simulink model "fboard_dwgn"  (Simulink 6.2)
settings: Solver=FixedStepDiscrete  SolverMode=SingleTasking  StartTime=0.0  StopTime=10.0  FixedStep=1  RelTol=1e-3
undefined symbols (not defined in the file): quant
libraries: xbsIndex_r3 x212, fb_xaui x1
(part 2 of 2)

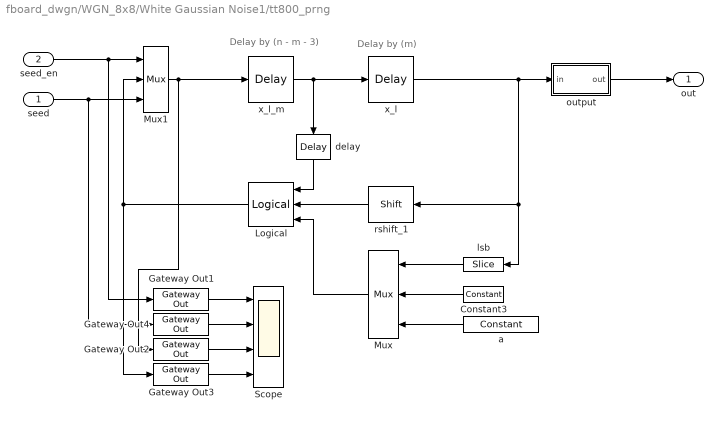
== system fboard_dwgn/WGN_8x8/White Gaussian Noise1/tt800_prng ==
  note: Delay by (n - m - 3)
  note: Delay by (m)
  seed : Inport  Port=1  LatchInput=off
  seed_en : Inport  Port=2  LatchInput=off
  Constant3 : xbsIndex_r3/Constant  Orientation=left  const=0  equ=P=C  arith_type=Unsigned  n_bits=32  bin_pt=0  opselect=C  inp2=PCIN>>17  opr=+  inp1=P  carry=CIN  iostate=0  explicit_period=off  period=1  dbl_ovrd=off
  Gateway Out{1..4} (4 alike) : xbsIndex_r3/Gateway Out  output_type=Double  nbits=8  bin_pt=6  arith_type=Boolean  quantization=Truncate  overflow=Wrap  hdl_port=off  timing_constraint=None  locs_specified=off  LOCs={}  needs_fixed_name=off  show_param=off
      settings: xl_area=[0 0 0 0 0 0 0]
  Logical : xbsIndex_r3/Logical  Orientation=left  logical_function=XOR  inputs=3  precision=Full  arith_type=Unsigned  n_bits=8  bin_pt=2  align_bp=off  latency=1  explicit_period=off  period=1  en=off  dbl_ovrd=off  show_param=on
      settings: xl_area=[32 32 0 32 0 0 0]
  Mux : xbsIndex_r3/Mux  Orientation=left  inputs=2  precision=Full  arith_type="Signed  (2's comp)"  n_bits=8  bin_pt=2  quantization=Truncate  overflow=Wrap  latency=1  explicit_period=off  period=1  en=off  dbl_ovrd=off  show_param=off  mux_type=off  use_rpm=off  gen_core=off
      settings: xl_area=[16 32 0 32 0 0 0]
  Mux1 : xbsIndex_r3/Mux  inputs=2  precision=Full  arith_type="Signed  (2's comp)"  n_bits=8  bin_pt=2  quantization=Truncate  overflow=Wrap  latency=1  explicit_period=on  period=1  en=off  dbl_ovrd=off  show_param=on  mux_type=off  use_rpm=off  gen_core=off
      settings: xl_area=[16 32 0 32 0 0 0]
  Scope : Scope  NumInputPorts=4
      settings: YMin=-5~-5~-5~-5  YMax=5~5~5~5
  a : xbsIndex_r3/Constant  Orientation=left  const=hex2dec('8EBFD028')  equ=P=C  arith_type=Unsigned  n_bits=32  bin_pt=0  opselect=C  inp2=PCIN>>17  opr=+  inp1=P  carry=CIN  iostate=0  explicit_period=off  period=1  dbl_ovrd=off
  delay : xbsIndex_r3/Delay  Orientation=down  latency=1  reg_retiming=off  explicit_period=off  period=1  en=off  accept_only_valid=off  init_zero=on  dbl_ovrd=off  show_param=off
      settings: xl_area=[16 32 0 0 0 0 0]
  lsb : xbsIndex_r3/Slice  Orientation=left  mode=Lower Bit Location + Width  nbits=1  bit1=0  base1=MSB of Input  bit0=0  base0=LSB of Input  boolean_output=off  explicit_period=off  period=1  dbl_ovrd=off
  output : Subsystem
  rshift_1 : xbsIndex_r3/Shift  Orientation=left  shift_dir=Right  shift_bits=1  precision=User Defined  arith_type=Unsigned  n_bits=32  bin_pt=0  quantization=Truncate  overflow=Wrap  latency=1  explicit_period=off  period=1  en=off  dbl_ovrd=off  show_param=off
      settings: xl_area=[0 32 0 0 0 0 0]
  x_l : xbsIndex_r3/Delay  latency=7  reg_retiming=off  explicit_period=off  period=1  en=off  accept_only_valid=off  init_zero=on  dbl_ovrd=off  show_param=off
      settings: xl_area=[16 32 0 32 0 0 0]
  x_l_m : xbsIndex_r3/Delay  latency=25-7-3  reg_retiming=off  explicit_period=off  period=1  en=off  accept_only_valid=off  init_zero=on  dbl_ovrd=off  show_param=off
      settings: xl_area=[16 32 0 32 0 0 0]
  out : Outport
  wires:
  delay/1 -> Logical/1
  output/1(out) -> out/1
  Gateway Out3/1 -> Scope/4
  Gateway Out2/1 -> Scope/3
  Gateway Out4/1 -> Scope/2
  Gateway Out1/1 -> Scope/1
  seed/1 -> Mux1/3, Gateway Out4/1
  seed_en/1 -> Mux1/1, Gateway Out1/1
  Mux1/1 -> Gateway Out2/1, x_l_m/1
  Logical/1 -> Mux1/2, Gateway Out3/1
  Mux/1 -> Logical/3
  rshift_1/1 -> Logical/2
  a/1 -> Mux/3
  Constant3/1 -> Mux/2
  lsb/1 -> Mux/1
  x_l/1 -> output/1(in), rshift_1/1, lsb/1
  x_l_m/1 -> delay/1, x_l/1

== system fboard_dwgn/WGN_8x8/White Gaussian Noise1/tt800_seed_gen ==
  seed_in : Inport  Port=1  LatchInput=off
  ld : Inport  Port=2  LatchInput=off
  Expression : xbsIndex_r3/Expression  expression=ld | ld_ext  precision=Full  arith_type=Unsigned  n_bits=8  bin_pt=2  align_bp=on  latency=1  explicit_period=off  period=1  en=off  dbl_ovrd=off  show_param=on
      settings: xl_area=[0, 0, 0, 0, 0, 0, 0]
  LFSR : xbsIndex_r3/LFSR  lfsr_type=Fibonacci  gate_type=XOR  output_type=on  n_bits=32  bin_pt=0  arith_type=Unsigned  polynomial='C0000401'  rst_value=dec2hex(seed)  reloadable_seed=on  input_type=on  explicit_period=on  period=1  rst=off  en=off  dbl_ovrd=off  show_param=on  useSRL16s=off  use_rpm=off  gen_core=off
      settings: xl_area=[17 32 0 33 0 0 0]
  p24_extender : Subsystem
  r_edge_detect : Subsystem
  seed_out : Outport
  seed_en : Outport  Port=2
  wires:
  r_edge_detect/1(out) -> p24_extender/1(in)
  p24_extender/1(out) -> Expression/2
  ld/1 -> LFSR/2, r_edge_detect/1(in), Expression/1
  Expression/1 -> seed_en/1
  seed_in/1 -> LFSR/1
  LFSR/1 -> seed_out/1

== system fboard_dwgn/WGN_8x8/White Gaussian Noise1/u2n ==
  u : Inport  Port=1  LatchInput=off
  Gateway Out : xbsIndex_r3/Gateway Out  output_type=Double  nbits=8  bin_pt=6  arith_type=Boolean  quantization=Truncate  overflow=Wrap  hdl_port=off  timing_constraint=None  locs_specified=off  LOCs={}  needs_fixed_name=off  show_param=off
      settings: xl_area=[0 0 0 0 17 0 0]
  Gateway Out1 : xbsIndex_r3/Gateway Out  output_type=Double  nbits=8  bin_pt=6  arith_type=Boolean  quantization=Truncate  overflow=Wrap  hdl_port=off  timing_constraint=None  locs_specified=off  LOCs={}  needs_fixed_name=off  show_param=off
      settings: xl_area=[0 0 0 0 17 0 0]
  Scope : Scope  NumInputPorts=2
      settings: YMin=-5~-5  YMax=5~5
  SineCosine : xbsIndex_r3/SineCosine  mode=Sine and Cosine  neg_sin=off  neg_cos=off  n_bits=8  latency=2  sym_output=off  explicit_period=off  period=1  en=off  dbl_ovrd=off  show_param=on  mem_type=Block RAM  pipeline=on  use_rpm=on  gen_core=off
      settings: xl_area=[8 16 1 2 0 0 0]
  bottom_11 : xbsIndex_r3/Slice  mode=Lower Bit Location + Width  nbits=11  bit1=0  base1=MSB of Input  bit0=0  base0=LSB of Input  boolean_output=off  explicit_period=off  period=1  dbl_ovrd=off
  log_lut : xbsIndex_r3/ROM  depth=2^11  initVector=quant(sqrt(-2*log(linspace(2^-11,1,2^11))),2^-7)  arith_type=Unsigned  n_bits=9  bin_pt=7  latency=1  init_zero=on  explicit_period=off  period=1  rst=off  init_reg=0  en=off  dbl_ovrd=off  show_param=off  distributed_mem=off  use_rpm=off  gen_core=off
      settings: xl_area=[0 0 1 0 0 0 0]
  r_cos : xbsIndex_r3/Mult  precision=Full  arith_type="Signed  (2's comp)"  n_bits=8  bin_pt=2  quantization=Truncate  overflow=Wrap  latency=3  explicit_period=off  period=1  en=off  dbl_ovrd=off  show_param=on  mult_type=Parallel  oversample=2  use_embedded=on  pipeline=on  use_rpm=on  placement_style=Rectangular Shape  gen_core=off
      settings: xl_area=[18 34 0 17 0 1 0]
  r_sin : xbsIndex_r3/Mult  precision=Full  arith_type="Signed  (2's comp)"  n_bits=8  bin_pt=2  quantization=Truncate  overflow=Wrap  latency=3  explicit_period=off  period=1  en=off  dbl_ovrd=off  show_param=on  mult_type=Parallel  oversample=2  use_embedded=on  pipeline=on  use_rpm=on  placement_style=Rectangular Shape  gen_core=off
      settings: xl_area=[18 34 0 17 0 1 0]
  top_11 : xbsIndex_r3/Slice  mode=Upper Bit Location + Width  nbits=11  bit1=0  base1=MSB of Input  bit0=0  base0=MSB of Input  boolean_output=off  explicit_period=off  period=1  dbl_ovrd=off
  n1 : Outport
  n2 : Outport  Port=2
  wires:
  Gateway Out/1 -> Scope/1
  Gateway Out1/1 -> Scope/2
  bottom_11/1 -> SineCosine/1
  top_11/1 -> log_lut/1
  u/1 -> top_11/1, bottom_11/1
  SineCosine/2 -> r_cos/2
  log_lut/1 -> r_sin/1, r_cos/1
  SineCosine/1 -> r_sin/2
  r_sin/1 -> Gateway Out/1, n1/1
  r_cos/1 -> Gateway Out1/1, n2/1

== system fboard_dwgn/WGN_8x8/concat0/ri_to_c ==
  re : Inport  Port=1  LatchInput=off
  im : Inport  Port=2  LatchInput=off
  concat : xbsIndex_r3/Concat  num_inputs=2  explicit_period=off  period=1  dbl_ovrd=off
  force_im : xbsIndex_r3/Reinterpret  force_arith_type=on  arith_type=Unsigned  force_bin_pt=on  bin_pt=0  force_valid=on
  force_re : xbsIndex_r3/Reinterpret  force_arith_type=on  arith_type=Unsigned  force_bin_pt=on  bin_pt=0  force_valid=on
  c : Outport
  wires:
  force_re/1 -> concat/1
  force_im/1 -> concat/2
  re/1 -> force_re/1
  concat/1 -> c/1
  im/1 -> force_im/1

== system fboard_dwgn/WGN_8x8/concat0/ri_to_c1 ==
  re : Inport  Port=1  LatchInput=off
  im : Inport  Port=2  LatchInput=off
  concat : xbsIndex_r3/Concat  num_inputs=2  explicit_period=off  period=1  dbl_ovrd=off
  force_im : xbsIndex_r3/Reinterpret  force_arith_type=on  arith_type=Unsigned  force_bin_pt=on  bin_pt=0  force_valid=on
  force_re : xbsIndex_r3/Reinterpret  force_arith_type=on  arith_type=Unsigned  force_bin_pt=on  bin_pt=0  force_valid=on
  c : Outport
  wires:
  im/1 -> force_im/1
  concat/1 -> c/1
  re/1 -> force_re/1
  force_im/1 -> concat/2
  force_re/1 -> concat/1

== system fboard_dwgn/WGN_8x8/concat0/ri_to_c2 ==
  re : Inport  Port=1  LatchInput=off
  im : Inport  Port=2  LatchInput=off
  concat : xbsIndex_r3/Concat  num_inputs=2  explicit_period=off  period=1  dbl_ovrd=off
  force_im : xbsIndex_r3/Reinterpret  force_arith_type=on  arith_type=Unsigned  force_bin_pt=on  bin_pt=0  force_valid=on
  force_re : xbsIndex_r3/Reinterpret  force_arith_type=on  arith_type=Unsigned  force_bin_pt=on  bin_pt=0  force_valid=on
  c : Outport
  wires:
  force_re/1 -> concat/1
  force_im/1 -> concat/2
  re/1 -> force_re/1
  concat/1 -> c/1
  im/1 -> force_im/1

== system fboard_dwgn/pfb8/fir8/pfb_fir_0 ==
  pol1_in : Inport  Port=1  LatchInput=off
  pol2_in : Inport  Port=2  LatchInput=off
  sync_in : Inport  Port=3  LatchInput=off
  pfb_fir : xbsIndex_r3/Black Box  init_code=pfb_fir_config  sim_method=Inactive  show_param=off
      settings: xl_area=[0, 0, 0, 0, 0, 0, 0]
  pol1_out : Outport
  pol2_out : Outport  Port=2
  sync_out : Outport  Port=3
  wires:
  pol1_in/1 -> pfb_fir/1
  pfb_fir/1 -> pol1_out/1
  pol2_in/1 -> pfb_fir/2
  pfb_fir/2 -> pol2_out/1
  sync_in/1 -> pfb_fir/3
  pfb_fir/3 -> sync_out/1

== system fboard_dwgn/pfb8/fir8/pfb_fir_1 ==
  pol1_in : Inport  Port=1  LatchInput=off
  pol2_in : Inport  Port=2  LatchInput=off
  sync_in : Inport  Port=3  LatchInput=off
  pfb_fir : xbsIndex_r3/Black Box  init_code=pfb_fir_config  sim_method=Inactive  show_param=off
      settings: xl_area=[0, 0, 0, 0, 0, 0, 0]
  pol1_out : Outport
  pol2_out : Outport  Port=2
  sync_out : Outport  Port=3
  wires:
  pfb_fir/3 -> sync_out/1
  sync_in/1 -> pfb_fir/3
  pfb_fir/2 -> pol2_out/1
  pol2_in/1 -> pfb_fir/2
  pfb_fir/1 -> pol1_out/1
  pol1_in/1 -> pfb_fir/1

== system fboard_dwgn/pfb8/pfb_fft8/quadplex_fft_0 ==
  in0 : Inport  Port=1  LatchInput=off
  in1 : Inport  Port=2  LatchInput=off
  in2 : Inport  Port=3  LatchInput=off
  in3 : Inport  Port=4  LatchInput=off
  sync_in : Inport  Port=5  LatchInput=off
  pfb_fft : xbsIndex_r3/Black Box  init_code=pfb_fft_config  sim_method=Inactive  show_param=off
      settings: xl_area=[0, 0, 0, 0, 0, 0, 0]
  out0 : Outport
  out1 : Outport  Port=2
  out2 : Outport  Port=3
  out3 : Outport  Port=4
  sync_out : Outport  Port=5
  wires:
  in0/1 -> pfb_fft/1
  pfb_fft/1 -> out0/1
  in1/1 -> pfb_fft/2
  pfb_fft/2 -> out1/1
  in2/1 -> pfb_fft/3
  pfb_fft/3 -> out2/1
  in3/1 -> pfb_fft/4
  pfb_fft/4 -> out3/1
  sync_in/1 -> pfb_fft/5
  pfb_fft/5 -> sync_out/1

== system fboard_dwgn/xaui/status_monitor/bot_status_reformat ==
  in : Inport  Port=1  LatchInput=off
  Concat : xbsIndex_r3/Concat  num_inputs=4  explicit_period=off  period=1  dbl_ovrd=off
  aligned : xbsIndex_r3/Slice  mode=Lower Bit Location + Width  nbits=1  bit1=12  base1=MSB of Input  bit0=10  base0=LSB of Input  boolean_output=off  explicit_period=off  period=1  dbl_ovrd=off
  four_bits{1..4} (4 alike) : xbsIndex_r3/Convert  arith_type=Unsigned  n_bits=4  bin_pt=0  quantization=Truncate  overflow=Wrap  latency=0  explicit_period=off  period=1  dbl_ovrd=off  show_param=off  inserted_by_tool=off  pipeline=off
      settings: xl_area=[0, 0, 0, 0, 0, 0, 0]
  fsm : xbsIndex_r3/Slice  mode=Lower Bit Location + Width  nbits=4  bit1=12  base1=MSB of Input  bit0=0  base0=LSB of Input  boolean_output=off  explicit_period=off  period=1  dbl_ovrd=off
  link : xbsIndex_r3/Slice  mode=Lower Bit Location + Width  nbits=1  bit1=12  base1=MSB of Input  bit0=12  base0=LSB of Input  boolean_output=off  explicit_period=off  period=1  dbl_ovrd=off
  syncs : xbsIndex_r3/Slice  mode=Lower Bit Location + Width  nbits=4  bit1=12  base1=MSB of Input  bit0=6  base0=LSB of Input  boolean_output=off  explicit_period=off  period=1  dbl_ovrd=off
  out : Outport
  wires:
  in/1 -> syncs/1, fsm/1, aligned/1, link/1
  Concat/1 -> out/1
  four_bits4/1 -> Concat/4
  four_bits3/1 -> Concat/3
  four_bits2/1 -> Concat/2
  four_bits1/1 -> Concat/1
  fsm/1 -> four_bits4/1
  syncs/1 -> four_bits3/1
  aligned/1 -> four_bits2/1
  link/1 -> four_bits1/1

== system fboard_dwgn/xaui/status_monitor/top_status_reformat ==
  in : Inport  Port=1  LatchInput=off
  Concat : xbsIndex_r3/Concat  num_inputs=4  explicit_period=off  period=1  dbl_ovrd=off
  aligned : xbsIndex_r3/Slice  mode=Lower Bit Location + Width  nbits=1  bit1=12  base1=MSB of Input  bit0=10  base0=LSB of Input  boolean_output=off  explicit_period=off  period=1  dbl_ovrd=off
  four_bits{1..4} (4 alike) : xbsIndex_r3/Convert  arith_type=Unsigned  n_bits=4  bin_pt=0  quantization=Truncate  overflow=Wrap  latency=0  explicit_period=off  period=1  dbl_ovrd=off  show_param=off  inserted_by_tool=off  pipeline=off
      settings: xl_area=[0, 0, 0, 0, 0, 0, 0]
  fsm : xbsIndex_r3/Slice  mode=Lower Bit Location + Width  nbits=4  bit1=12  base1=MSB of Input  bit0=0  base0=LSB of Input  boolean_output=off  explicit_period=off  period=1  dbl_ovrd=off
  link : xbsIndex_r3/Slice  mode=Lower Bit Location + Width  nbits=1  bit1=12  base1=MSB of Input  bit0=12  base0=LSB of Input  boolean_output=off  explicit_period=off  period=1  dbl_ovrd=off
  syncs : xbsIndex_r3/Slice  mode=Lower Bit Location + Width  nbits=4  bit1=12  base1=MSB of Input  bit0=6  base0=LSB of Input  boolean_output=off  explicit_period=off  period=1  dbl_ovrd=off
  out : Outport
  wires:
  link/1 -> four_bits1/1
  aligned/1 -> four_bits2/1
  syncs/1 -> four_bits3/1
  fsm/1 -> four_bits4/1
  four_bits1/1 -> Concat/1
  four_bits2/1 -> Concat/2
  four_bits3/1 -> Concat/3
  four_bits4/1 -> Concat/4
  Concat/1 -> out/1
  in/1 -> link/1, aligned/1, fsm/1, syncs/1

== system fboard_dwgn/WGN_8x8/White Gaussian Noise/tt800_prng/output ==
  in : Inport  Port=1  LatchInput=off
  Logical1 : xbsIndex_r3/Logical  logical_function=XOR  inputs=2  precision=Full  arith_type=Unsigned  n_bits=8  bin_pt=2  align_bp=off  latency=1  explicit_period=off  period=1  en=off  dbl_ovrd=off  show_param=on
      settings: xl_area=[32 32 0 32 0 0 0]
  Logical2 : xbsIndex_r3/Logical  logical_function=XOR  inputs=2  precision=Full  arith_type=Unsigned  n_bits=8  bin_pt=2  align_bp=off  latency=1  explicit_period=off  period=1  en=off  dbl_ovrd=off  show_param=on
      settings: xl_area=[32 32 0 32 0 0 0]
  Logical3 : xbsIndex_r3/Logical  logical_function=AND  inputs=2  precision=Full  arith_type=Unsigned  n_bits=8  bin_pt=2  align_bp=off  latency=1  explicit_period=off  period=1  en=off  dbl_ovrd=off  show_param=on
      settings: xl_area=[32 32 0 32 0 0 0]
  Logical4 : xbsIndex_r3/Logical  logical_function=AND  inputs=2  precision=Full  arith_type=Unsigned  n_bits=8  bin_pt=2  align_bp=off  latency=1  explicit_period=off  period=1  en=off  dbl_ovrd=off  show_param=on
      settings: xl_area=[32 32 0 32 0 0 0]
  b : xbsIndex_r3/Constant  const=hex2dec('2B5B2500')  equ=P=C  arith_type=Unsigned  n_bits=32  bin_pt=0  opselect=C  inp2=PCIN>>17  opr=+  inp1=P  carry=CIN  iostate=0  explicit_period=off  period=1  dbl_ovrd=off
  c : xbsIndex_r3/Constant  const=hex2dec('DB8B0000')  equ=P=C  arith_type=Unsigned  n_bits=32  bin_pt=0  opselect=C  inp2=PCIN>>17  opr=+  inp1=P  carry=CIN  iostate=0  explicit_period=off  period=1  dbl_ovrd=off
  delay : xbsIndex_r3/Delay  latency=1  reg_retiming=off  explicit_period=off  period=1  en=off  accept_only_valid=off  init_zero=on  dbl_ovrd=off  show_param=off
      settings: xl_area=[16 32 0 0 0 0 0]
  delay1 : xbsIndex_r3/Delay  latency=1  reg_retiming=off  explicit_period=off  period=1  en=off  accept_only_valid=off  init_zero=on  dbl_ovrd=off  show_param=off
      settings: xl_area=[16 32 0 0 0 0 0]
  lshift_s : xbsIndex_r3/Shift  shift_dir=Left  shift_bits=7  precision=User Defined  arith_type=Unsigned  n_bits=32  bin_pt=0  quantization=Truncate  overflow=Wrap  latency=0  explicit_period=off  period=1  en=off  dbl_ovrd=off  show_param=off
      settings: xl_area=[0 0 0 0 0 0 0]
  lshift_t : xbsIndex_r3/Shift  shift_dir=Left  shift_bits=15  precision=User Defined  arith_type=Unsigned  n_bits=32  bin_pt=0  quantization=Truncate  overflow=Wrap  latency=0  explicit_period=off  period=1  en=off  dbl_ovrd=off  show_param=off
      settings: xl_area=[0 0 0 0 0 0 0]
  out : Outport
  wires:
  Logical2/1 -> out/1
  in/1 -> lshift_s/1, delay/1
  Logical4/1 -> Logical2/2
  delay1/1 -> Logical2/1
  c/1 -> Logical4/2
  lshift_t/1 -> Logical4/1
  Logical1/1 -> lshift_t/1, delay1/1
  Logical3/1 -> Logical1/2
  b/1 -> Logical3/2
  lshift_s/1 -> Logical3/1
  delay/1 -> Logical1/1

== system fboard_dwgn/WGN_8x8/White Gaussian Noise/tt800_seed_gen/p24_extender ==
  in : Inport  Port=1  LatchInput=off
  Constant3 : xbsIndex_r3/Constant  const=1  equ=P=C  arith_type=Boolean  n_bits=1  bin_pt=0  opselect=C  inp2=PCIN>>17  opr=+  inp1=P  carry=CIN  iostate=0  explicit_period=on  period=1  dbl_ovrd=off
  Delay : xbsIndex_r3/Delay  latency=24  reg_retiming=off  explicit_period=off  period=1  en=off  accept_only_valid=off  init_zero=on  dbl_ovrd=off  show_param=off
      settings: xl_area=[2 2 0 2 0 0 0]
  Register : xbsIndex_r3/Register  init=0  reg_only_valid=off  explicit_period=off  period=1  rst=on  en=on  out_en=off  dbl_ovrd=off  show_param=on
      settings: xl_area=[1 1 0 0 0 0 0]
  out : Outport
  wires:
  in/1 -> Delay/1, Register/3
  Delay/1 -> Register/2
  Constant3/1 -> Register/1
  Register/1 -> out/1

== system fboard_dwgn/WGN_8x8/White Gaussian Noise/tt800_seed_gen/r_edge_detect ==
  in : Inport  Port=1  LatchInput=off
  Delay : xbsIndex_r3/Delay  latency=1  reg_retiming=off  explicit_period=off  period=1  en=off  accept_only_valid=off  init_zero=on  dbl_ovrd=off  show_param=off
      settings: xl_area=[1 1 0 0 0 0 0]
  Expression : xbsIndex_r3/Expression  expression=curr & ~prev  precision=Full  arith_type=Unsigned  n_bits=8  bin_pt=2  align_bp=on  latency=0  explicit_period=off  period=1  en=off  dbl_ovrd=off  show_param=off
      settings: xl_area=[0, 0, 0, 0, 0, 0, 0]
  out : Outport
  wires:
  in/1 -> Expression/1, Delay/1
  Delay/1 -> Expression/2
  Expression/1 -> out/1

== system fboard_dwgn/WGN_8x8/White Gaussian Noise1/tt800_prng/output ==
  in : Inport  Port=1  LatchInput=off
  Logical1 : xbsIndex_r3/Logical  logical_function=XOR  inputs=2  precision=Full  arith_type=Unsigned  n_bits=8  bin_pt=2  align_bp=off  latency=1  explicit_period=off  period=1  en=off  dbl_ovrd=off  show_param=on
      settings: xl_area=[32 32 0 32 0 0 0]
  Logical2 : xbsIndex_r3/Logical  logical_function=XOR  inputs=2  precision=Full  arith_type=Unsigned  n_bits=8  bin_pt=2  align_bp=off  latency=1  explicit_period=off  period=1  en=off  dbl_ovrd=off  show_param=on
      settings: xl_area=[32 32 0 32 0 0 0]
  Logical3 : xbsIndex_r3/Logical  logical_function=AND  inputs=2  precision=Full  arith_type=Unsigned  n_bits=8  bin_pt=2  align_bp=off  latency=1  explicit_period=off  period=1  en=off  dbl_ovrd=off  show_param=on
      settings: xl_area=[32 32 0 32 0 0 0]
  Logical4 : xbsIndex_r3/Logical  logical_function=AND  inputs=2  precision=Full  arith_type=Unsigned  n_bits=8  bin_pt=2  align_bp=off  latency=1  explicit_period=off  period=1  en=off  dbl_ovrd=off  show_param=on
      settings: xl_area=[32 32 0 32 0 0 0]
  b : xbsIndex_r3/Constant  const=hex2dec('2B5B2500')  equ=P=C  arith_type=Unsigned  n_bits=32  bin_pt=0  opselect=C  inp2=PCIN>>17  opr=+  inp1=P  carry=CIN  iostate=0  explicit_period=off  period=1  dbl_ovrd=off
  c : xbsIndex_r3/Constant  const=hex2dec('DB8B0000')  equ=P=C  arith_type=Unsigned  n_bits=32  bin_pt=0  opselect=C  inp2=PCIN>>17  opr=+  inp1=P  carry=CIN  iostate=0  explicit_period=off  period=1  dbl_ovrd=off
  delay : xbsIndex_r3/Delay  latency=1  reg_retiming=off  explicit_period=off  period=1  en=off  accept_only_valid=off  init_zero=on  dbl_ovrd=off  show_param=off
      settings: xl_area=[16 32 0 0 0 0 0]
  delay1 : xbsIndex_r3/Delay  latency=1  reg_retiming=off  explicit_period=off  period=1  en=off  accept_only_valid=off  init_zero=on  dbl_ovrd=off  show_param=off
      settings: xl_area=[16 32 0 0 0 0 0]
  lshift_s : xbsIndex_r3/Shift  shift_dir=Left  shift_bits=7  precision=User Defined  arith_type=Unsigned  n_bits=32  bin_pt=0  quantization=Truncate  overflow=Wrap  latency=0  explicit_period=off  period=1  en=off  dbl_ovrd=off  show_param=off
      settings: xl_area=[0 0 0 0 0 0 0]
  lshift_t : xbsIndex_r3/Shift  shift_dir=Left  shift_bits=15  precision=User Defined  arith_type=Unsigned  n_bits=32  bin_pt=0  quantization=Truncate  overflow=Wrap  latency=0  explicit_period=off  period=1  en=off  dbl_ovrd=off  show_param=off
      settings: xl_area=[0 0 0 0 0 0 0]
  out : Outport
  wires:
  Logical2/1 -> out/1
  in/1 -> lshift_s/1, delay/1
  Logical4/1 -> Logical2/2
  delay1/1 -> Logical2/1
  c/1 -> Logical4/2
  lshift_t/1 -> Logical4/1
  Logical1/1 -> lshift_t/1, delay1/1
  Logical3/1 -> Logical1/2
  b/1 -> Logical3/2
  lshift_s/1 -> Logical3/1
  delay/1 -> Logical1/1

== system fboard_dwgn/WGN_8x8/White Gaussian Noise1/tt800_seed_gen/p24_extender ==
  in : Inport  Port=1  LatchInput=off
  Constant3 : xbsIndex_r3/Constant  const=1  equ=P=C  arith_type=Boolean  n_bits=1  bin_pt=0  opselect=C  inp2=PCIN>>17  opr=+  inp1=P  carry=CIN  iostate=0  explicit_period=on  period=1  dbl_ovrd=off
  Delay : xbsIndex_r3/Delay  latency=24  reg_retiming=off  explicit_period=off  period=1  en=off  accept_only_valid=off  init_zero=on  dbl_ovrd=off  show_param=off
      settings: xl_area=[2 2 0 2 0 0 0]
  Register : xbsIndex_r3/Register  init=0  reg_only_valid=off  explicit_period=off  period=1  rst=on  en=on  out_en=off  dbl_ovrd=off  show_param=on
      settings: xl_area=[1 1 0 0 0 0 0]
  out : Outport
  wires:
  in/1 -> Delay/1, Register/3
  Delay/1 -> Register/2
  Constant3/1 -> Register/1
  Register/1 -> out/1

== system fboard_dwgn/WGN_8x8/White Gaussian Noise1/tt800_seed_gen/r_edge_detect ==
  in : Inport  Port=1  LatchInput=off
  Delay : xbsIndex_r3/Delay  latency=1  reg_retiming=off  explicit_period=off  period=1  en=off  accept_only_valid=off  init_zero=on  dbl_ovrd=off  show_param=off
      settings: xl_area=[1 1 0 0 0 0 0]
  Expression : xbsIndex_r3/Expression  expression=curr & ~prev  precision=Full  arith_type=Unsigned  n_bits=8  bin_pt=2  align_bp=on  latency=0  explicit_period=off  period=1  en=off  dbl_ovrd=off  show_param=off
      settings: xl_area=[0, 0, 0, 0, 0, 0, 0]
  out : Outport
  wires:
  in/1 -> Expression/1, Delay/1
  Delay/1 -> Expression/2
  Expression/1 -> out/1
